simulink model "IEEE34_PQload"  (R2021b)
settings: Solver=ode4  StartTime=0.0  StopTime=5  FixedStep=50e-6  RelTol=1e-3
PreLoadFcn:
  | pGain = 0.05; % Gain of random perturbation (pu)
  | pGainAP = 0.01; % Gain of sinusoidal active power variation (pu)
  | pGainRP = 0.01; % Gain of sinusoidal reactive power variation (pu)
  | pFreqAP = 0.03; % Frequency of sinusoidal active power variation (Hz)
  | pFreqRP = 0.03; % Frequency of sinusoidal reactive power variation (Hz)
  | 
  | init_IEEE34nodetestfeeder;
InitFcn:
  | pGain = 0.05; % Gain of random perturbation (pu)
  | pGainAP = 0.01; % Gain of sinusoidal active power variation (pu)
  | pGainRP = 0.01; % Gain of sinusoidal reactive power variation (pu)
  | pFreqAP = 0.03; % Frequency of sinusoidal active power variation (Hz)
  | pFreqRP = 0.03; % Frequency of sinusoidal reactive power variation (Hz)
  | 
  | init_IEEE34nodetestfeeder;
values from neighbouring files (symbols this model uses):
  fNom = f    (= 60)    [init_IEEE34nodetestfeeder.m]
  loadcoeff = 1.0    (= 1)    [init_IEEE34nodetestfeeder.m]
  Pbase = 500e3    (= 500000)    [init_IEEE34nodetestfeeder.m]
  Ts = 50e-6    (= 5e-05)    [init_IEEE34nodetestfeeder.m]
  vNomMV = VsubL    (= 24900)    [init_IEEE34nodetestfeeder.m]
  VsubL = 24.9e3    (= 24900)    [init_IEEE34nodetestfeeder.m]
undefined symbols (not defined in the file or in its folder): find_system
libraries: spsSeriesRLCBranchLib x330, spsGroundLib x242, LoadLib x88, spsThreePhaseVIMeasurementLib x37, spsMutualInductanceLib x24, spsVoltageMeasurementLib x18, spsCurrentMeasurementLib x12, spsOnDelayLib x12, spsRMSLib x8, spsLinearTransformerLib x6, spsControlledCurrentSourceLib x6, spsControlledVoltageSourceLib x6
(part 6 of 8)

== system IEEE34_PQload/SM_IEEE34/Regulator 2 ==
  Mux : Mux  Inputs=3
  Single Phase SVR_A : Subsystem  LoadFcn=find_system(gcs,'FollowLinks', 'on', 'LookUnderMasks', 'all');  mask(Single-Phase OLTC){pNom=5e6/3, fNom=60, vNom=24.9e3/sqrt(3), ctRatio=100, ptRatio=120, DeltaU=0.00625, TapMinMax=[-16 16], InitialTap=-13, TapSelectionTime=0.2, RegulatorOn=off, Regulator=[124/120  2/120  0.2], Comp=[2.5 1.5]}
      mask prompts: pNom "Nominal Power (VA)"; fNom "Nominal Frequency (Hz)"; vNom "Nominal Voltage (Vrms)"; ctRatio "Primary CT Rating (A)"; ptRatio "PT Ratio"; DeltaU "Voltage Step Per Tap (pu)"; TapMinMax "Minimum and Maximum Tap Positions"; InitialTap "Initial Tap Position"; TapSelectionTime "Tap Selection Time (s)"; RegulatorOn "Voltage Regulator"; Regulator "Voltage Regulator [ Vref(pu) DeadBand(pu)  Delay(s)]"; Comp "Compensator Settings [R (V) X(V)]"
      mask help:
      | Models a single-phase On Load Tap Changer (OLTC). The single-phase primary of multi-tap winding is modeled with a Variable-Ratio Transformer block.
      |
      | The transformer voltage ratio U2/U1 (in pu) is given by:
      |                 U2/U1= 1/ (1+TapPosition*DeltaU)
      | Tap position 0 corresponds to nominal voltage ratio.
      |
      | When Voltage regulator is 'on',  voltage regulator asks for a tap change if:
      |                  abs(Vm-Vref)>DeadBand/2  during a time  t > Delay.
      |
      | where 'Vm' is voltage measured at regulating point and Vref is reference voltage.
      | With line drop compensation, Vm=Vsec-Isec(R+jX)
      mask init:
      | RegulatorVref=Regulator(1);
      | RegulatorDeadBand=Regulator(2);
      | RegulatorDelay=Regulator(3);
      | Rc=Comp(1);
      | Xc=Comp(2);
      mask TypeOptions RegulatorOn: off | on
      mask Callback RegulatorOn:
      | tempMaskVis=get_param(gcb,'MaskVisibilities');
      | if strcmp(get_param(gcb,'RegulatorOn'),'on')
      | 	tempMaskVis{11}='on';
      | 	set_param(gcb,'MaskVisibilities',tempMaskVis);
      | else
      | 	tempMaskVis{11}='off';
      | 	set_param(gcb,'MaskVisibilities',tempMaskVis);
      | end
      | if strcmp(get_param(gcb,'RegulatorOn'),'on')
      | 	tempMaskVis{12}='on';
      | 	set_param(gcb,'MaskVisibilities',tempMaskVis);
      | else
      | 	tempMaskVis{12}='off';
      | 	set_param(gcb,'MaskVisibilities',tempMaskVis);
      | end
      mask DialogControl Container8 Prompt: Setup
      mask DialogControl Container13 Prompt: Regulator Parameters
  Single Phase SVR_B : Subsystem  LoadFcn=find_system(gcs,'FollowLinks', 'on', 'LookUnderMasks', 'all');  mask(Single-Phase OLTC){pNom=5e6/3, fNom=60, vNom=24.9e3/sqrt(3), ctRatio=100, ptRatio=120, DeltaU=0.00625, TapMinMax=[-16 16], InitialTap=-11, TapSelectionTime=0.2, RegulatorOn=off, Regulator=[124/120  2/120  0.2], Comp=[2.5 1.5]}
      mask prompts: pNom "Nominal Power (VA)"; fNom "Nominal Frequency (Hz)"; vNom "Nominal Voltage (Vrms)"; ctRatio "Primary CT Rating (A)"; ptRatio "PT Ratio"; DeltaU "Voltage Step Per Tap (pu)"; TapMinMax "Minimum and Maximum Tap Positions"; InitialTap "Initial Tap Position"; TapSelectionTime "Tap Selection Time (s)"; RegulatorOn "Voltage Regulator"; Regulator "Voltage Regulator [ Vref(pu) DeadBand(pu)  Delay(s)]"; Comp "Compensator Settings [R (V) X(V)]"
      mask help:
      | Models a single-phase On Load Tap Changer (OLTC). The single-phase primary of multi-tap winding is modeled with a Variable-Ratio Transformer block.
      |
      | The transformer voltage ratio U2/U1 (in pu) is given by:
      |                 U2/U1= 1/ (1+TapPosition*DeltaU)
      | Tap position 0 corresponds to nominal voltage ratio.
      |
      | When Voltage regulator is 'on',  voltage regulator asks for a tap change if:
      |                  abs(Vm-Vref)>DeadBand/2  during a time  t > Delay.
      |
      | where 'Vm' is voltage measured at regulating point and Vref is reference voltage.
      | With line drop compensation, Vm=Vsec-Isec(R+jX)
      mask init:
      | RegulatorVref=Regulator(1);
      | RegulatorDeadBand=Regulator(2);
      | RegulatorDelay=Regulator(3);
      | Rc=Comp(1);
      | Xc=Comp(2);
      mask TypeOptions RegulatorOn: off | on
      mask Callback RegulatorOn:
      | tempMaskVis=get_param(gcb,'MaskVisibilities');
      | if strcmp(get_param(gcb,'RegulatorOn'),'on')
      | 	tempMaskVis{11}='on';
      | 	set_param(gcb,'MaskVisibilities',tempMaskVis);
      | else
      | 	tempMaskVis{11}='off';
      | 	set_param(gcb,'MaskVisibilities',tempMaskVis);
      | end
      | if strcmp(get_param(gcb,'RegulatorOn'),'on')
      | 	tempMaskVis{12}='on';
      | 	set_param(gcb,'MaskVisibilities',tempMaskVis);
      | else
      | 	tempMaskVis{12}='off';
      | 	set_param(gcb,'MaskVisibilities',tempMaskVis);
      | end
      mask DialogControl Container8 Prompt: Setup
      mask DialogControl Container13 Prompt: Regulator Parameters
  Single Phase SVR_C : Subsystem  LoadFcn=find_system(gcs,'FollowLinks', 'on', 'LookUnderMasks', 'all');  mask(Single-Phase OLTC){pNom=5e6/3, fNom=60, vNom=24.9e3/sqrt(3), ctRatio=100, ptRatio=120, DeltaU=0.00625, TapMinMax=[-16 16], InitialTap=-12, TapSelectionTime=0.2, RegulatorOn=off, Regulator=[124/120  2/120  0.2], Comp=[2.5 1.5]}
      mask prompts: pNom "Nominal Power (VA)"; fNom "Nominal Frequency (Hz)"; vNom "Nominal Voltage (Vrms)"; ctRatio "Primary CT Rating (A)"; ptRatio "PT Ratio"; DeltaU "Voltage Step Per Tap (pu)"; TapMinMax "Minimum and Maximum Tap Positions"; InitialTap "Initial Tap Position"; TapSelectionTime "Tap Selection Time (s)"; RegulatorOn "Voltage Regulator"; Regulator "Voltage Regulator [ Vref(pu) DeadBand(pu)  Delay(s)]"; Comp "Compensator Settings [R (V) X(V)]"
      mask help:
      | Models a single-phase On Load Tap Changer (OLTC). The single-phase primary of multi-tap winding is modeled with a Variable-Ratio Transformer block.
      |
      | The transformer voltage ratio U2/U1 (in pu) is given by:
      |                 U2/U1= 1/ (1+TapPosition*DeltaU)
      | Tap position 0 corresponds to nominal voltage ratio.
      |
      | When Voltage regulator is 'on',  voltage regulator asks for a tap change if:
      |                  abs(Vm-Vref)>DeadBand/2  during a time  t > Delay.
      |
      | where 'Vm' is voltage measured at regulating point and Vref is reference voltage.
      | With line drop compensation, Vm=Vsec-Isec(R+jX)
      mask init:
      | RegulatorVref=Regulator(1);
      | RegulatorDeadBand=Regulator(2);
      | RegulatorDelay=Regulator(3);
      | Rc=Comp(1);
      | Xc=Comp(2);
      mask TypeOptions RegulatorOn: off | on
      mask Callback RegulatorOn:
      | tempMaskVis=get_param(gcb,'MaskVisibilities');
      | if strcmp(get_param(gcb,'RegulatorOn'),'on')
      | 	tempMaskVis{11}='on';
      | 	set_param(gcb,'MaskVisibilities',tempMaskVis);
      | else
      | 	tempMaskVis{11}='off';
      | 	set_param(gcb,'MaskVisibilities',tempMaskVis);
      | end
      | if strcmp(get_param(gcb,'RegulatorOn'),'on')
      | 	tempMaskVis{12}='on';
      | 	set_param(gcb,'MaskVisibilities',tempMaskVis);
      | else
      | 	tempMaskVis{12}='off';
      | 	set_param(gcb,'MaskVisibilities',tempMaskVis);
      | end
      mask DialogControl Container8 Prompt: Setup
      mask DialogControl Container13 Prompt: Regulator Parameters
  A : PMIOPort  Side=Left
  a : PMIOPort  Port=2  Side=Right
  B : PMIOPort  Port=3  Side=Left
  b : PMIOPort  Port=4  Side=Right
  C : PMIOPort  Port=5  Side=Left
  c : PMIOPort  Port=6  Side=Right
  Tap : Outport
  wires:
  Single Phase SVR_A/1(Tap) -> Mux/1
  Single Phase SVR_B/1(Tap) -> Mux/2
  Single Phase SVR_C/1(Tap) -> Mux/3
  Mux/1 -> Tap/1
  connections:
  Single Phase SVR_A/RConn1 -- a/RConn1
  Single Phase SVR_A/LConn1 -- A/RConn1
  Single Phase SVR_B/LConn1 -- B/RConn1
  Single Phase SVR_B/RConn1 -- b/RConn1
  Single Phase SVR_C/LConn1 -- C/RConn1
  Single Phase SVR_C/RConn1 -- c/RConn1

== system IEEE34_PQload/SM_IEEE34/Spot 830 ==
  SinglePhase_PQLoadwithFeedback : LoadLib/SinglePhase_PQLoad  fnom=60  Vbase=VsubL  V0=1  S0=[10*1000*loadcoeff 5*1000*loadcoeff]/Pbase  PQext=off  Kpi=PI_values  BasePower=Pbase  n=[2 2]  T=[0 0 0 0]  Vmin=0.7  Freq_dep=on  FKpq=[0 0]  Ts=50e-6
  SinglePhase_PQLoadwithFeedback1 : LoadLib/SinglePhase_PQLoad  fnom=60  Vbase=VsubL  V0=1  S0=[10*1000*loadcoeff 5*1000*loadcoeff]/Pbase  PQext=off  Kpi=PI_values  BasePower=Pbase  n=[2 2]  T=[0 0 0 0]  Vmin=0.7  Freq_dep=on  FKpq=[0 0]  Ts=50e-6
  SinglePhase_PQLoadwithFeedback2 : LoadLib/SinglePhase_PQLoad  fnom=60  Vbase=VsubL  V0=1  S0=[25*1000*loadcoeff 10*1000*loadcoeff]/Pbase  PQext=off  Kpi=PI_values  BasePower=Pbase  n=[2 2]  T=[0 0 0 0]  Vmin=0.7  Freq_dep=on  FKpq=[0 0]  Ts=50e-6
  Terminator3 : Terminator
  Terminator4 : Terminator
  Terminator5 : Terminator
  A : PMIOPort  Side=Right
  B : PMIOPort  Port=2  Side=Right
  C : PMIOPort  Port=3  Side=Right
  wires:
  SinglePhase_PQLoadwithFeedback/1 -> Terminator3/1
  SinglePhase_PQLoadwithFeedback1/1 -> Terminator4/1
  SinglePhase_PQLoadwithFeedback2/1 -> Terminator5/1
  connections:
  SinglePhase_PQLoadwithFeedback/LConn1 -- SinglePhase_PQLoadwithFeedback2/LConn2 -- A/RConn1
  SinglePhase_PQLoadwithFeedback1/LConn1 -- SinglePhase_PQLoadwithFeedback/LConn2 -- B/RConn1
  SinglePhase_PQLoadwithFeedback2/LConn1 -- SinglePhase_PQLoadwithFeedback1/LConn2 -- C/RConn1

== system IEEE34_PQload/SM_IEEE34/Spot 840 ==
  Ground1 : spsGroundLib/Ground  LConnTagsString=a
  Ground2 : spsGroundLib/Ground  LConnTagsString=a
  Ground3 : spsGroundLib/Ground  LConnTagsString=a
  SinglePhase_PQLoadwithFeedback : LoadLib/SinglePhase_PQLoad  fnom=60  Vbase=VsubL/sqrt(3)  V0=1  S0=[9*1000*loadcoeff 7*1000*loadcoeff]/Pbase  PQext=off  Kpi=PI_values  BasePower=Pbase  n=[1 1]  T=[0 0 0 0]  Vmin=0.7  Freq_dep=on  FKpq=[0 0]  Ts=50e-6
  SinglePhase_PQLoadwithFeedback1 : LoadLib/SinglePhase_PQLoad  fnom=60  Vbase=VsubL/sqrt(3)  V0=1  S0=[9*1000*loadcoeff 7*1000*loadcoeff]/Pbase  PQext=off  Kpi=PI_values  BasePower=Pbase  n=[1 1]  T=[0 0 0 0]  Vmin=0.7  Freq_dep=on  FKpq=[0 0]  Ts=50e-6
  SinglePhase_PQLoadwithFeedback2 : LoadLib/SinglePhase_PQLoad  fnom=60  Vbase=VsubL/sqrt(3)  V0=1  S0=[9*1000*loadcoeff 7*1000*loadcoeff]/Pbase  PQext=off  Kpi=PI_values  BasePower=Pbase  n=[1 1]  T=[0 0 0 0]  Vmin=0.7  Freq_dep=on  FKpq=[0 0]  Ts=50e-6
  Terminator3 : Terminator
  Terminator4 : Terminator
  Terminator5 : Terminator
  A : PMIOPort  Side=Right
  B : PMIOPort  Port=2  Side=Right
  C : PMIOPort  Port=3  Side=Right
  wires:
  SinglePhase_PQLoadwithFeedback/1 -> Terminator3/1
  SinglePhase_PQLoadwithFeedback1/1 -> Terminator4/1
  SinglePhase_PQLoadwithFeedback2/1 -> Terminator5/1
  connections:
  SinglePhase_PQLoadwithFeedback/LConn2 -- Ground1/LConn1
  SinglePhase_PQLoadwithFeedback1/LConn2 -- Ground2/LConn1
  SinglePhase_PQLoadwithFeedback2/LConn2 -- Ground3/LConn1
  SinglePhase_PQLoadwithFeedback/LConn1 -- A/RConn1
  SinglePhase_PQLoadwithFeedback1/LConn1 -- B/RConn1
  SinglePhase_PQLoadwithFeedback2/LConn1 -- C/RConn1

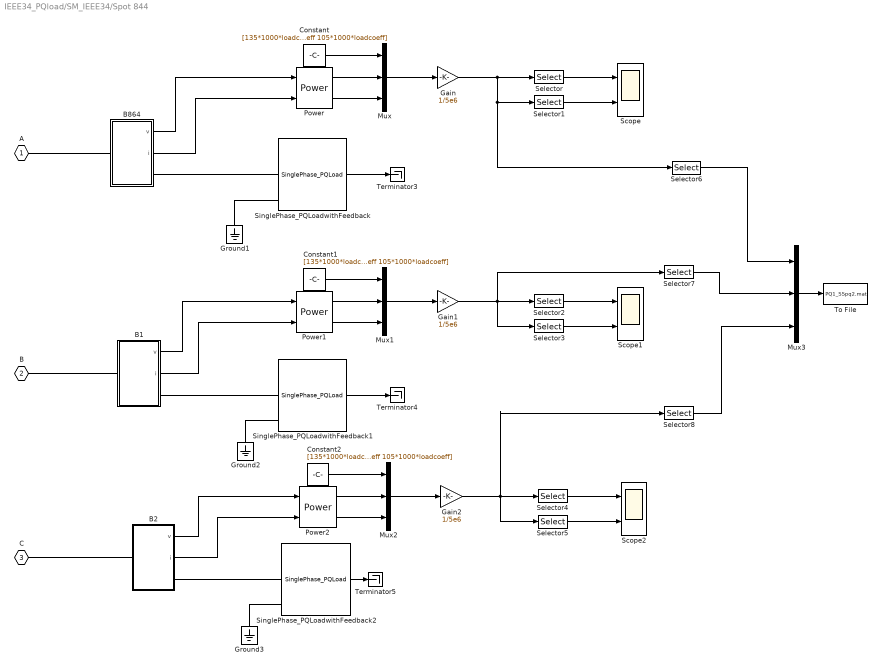
== system IEEE34_PQload/SM_IEEE34/Spot 844 ==
  B1 : Subsystem
  B2 : Subsystem
  B864 : Subsystem
  Constant : Constant  Value=[135*1000*loadcoeff 105*1000*loadcoeff]
  Constant1 : Constant  Value=[135*1000*loadcoeff 105*1000*loadcoeff]
  Constant2 : Constant  Value=[135*1000*loadcoeff 105*1000*loadcoeff]
  Gain : Gain  Gain=1/5e6
  Gain1 : Gain  Gain=1/5e6
  Gain2 : Gain  Gain=1/5e6
  Ground1 : spsGroundLib/Ground  LConnTagsString=a
  Ground2 : spsGroundLib/Ground  LConnTagsString=a
  Ground3 : spsGroundLib/Ground  LConnTagsString=a
  Mux{,1..3} (4 alike) : Mux  Inputs=3
  Power : spsPowerLib/Power  Freq=60  Vinit=[1, 0]  Iinit=[1, 0]  Ts=0
      settings: SourceProductBaseCode=PS
  Power1 : spsPowerLib/Power  Freq=60  Vinit=[1, 0]  Iinit=[1, 0]  Ts=0
      settings: SourceProductBaseCode=PS
  Power2 : spsPowerLib/Power  Freq=60  Vinit=[1, 0]  Iinit=[1, 0]  Ts=0
      settings: SourceProductBaseCode=PS
  Scope : Scope  NumInputPorts=2
  Scope1 : Scope  NumInputPorts=2
  Scope2 : Scope  NumInputPorts=2
  Selector : Selector  InputPortWidth=4  IndexOptions=Index vector (dialog)  Indices=[1 3]  OutputSizes=1
  Selector1 : Selector  InputPortWidth=4  IndexOptions=Index vector (dialog)  Indices=[2 4]  OutputSizes=1
  Selector2 : Selector  InputPortWidth=4  IndexOptions=Index vector (dialog)  Indices=[1 3]  OutputSizes=1
  Selector3 : Selector  InputPortWidth=4  IndexOptions=Index vector (dialog)  Indices=[2 4]  OutputSizes=1
  Selector4 : Selector  InputPortWidth=4  IndexOptions=Index vector (dialog)  Indices=[1 3]  OutputSizes=1
  Selector5 : Selector  InputPortWidth=4  IndexOptions=Index vector (dialog)  Indices=[2 4]  OutputSizes=1
  Selector6 : Selector  InputPortWidth=4  IndexOptions=Index vector (dialog)  Indices=[3 4]  OutputSizes=1
  Selector7 : Selector  InputPortWidth=4  IndexOptions=Index vector (dialog)  Indices=[3 4]  OutputSizes=1
  Selector8 : Selector  InputPortWidth=4  IndexOptions=Index vector (dialog)  Indices=[3 4]  OutputSizes=1
  SinglePhase_PQLoadwithFeedback : LoadLib/SinglePhase_PQLoad  fnom=60  Vbase=VsubL/sqrt(3)  V0=1  S0=[135*1000*loadcoeff 105*1000*loadcoeff]/Pbase  PQext=off  Kpi=PI_values  BasePower=Pbase  n=[2 2]  T=[0 0 0 0]  Vmin=0.7  Freq_dep=on  FKpq=[0 0]  Ts=50e-6
  SinglePhase_PQLoadwithFeedback1 : LoadLib/SinglePhase_PQLoad  fnom=60  Vbase=VsubL/sqrt(3)  V0=1  S0=[135*1000*loadcoeff 105*1000*loadcoeff]/Pbase  PQext=off  Kpi=PI_values  BasePower=Pbase  n=[2 2]  T=[0 0 0 0]  Vmin=0.7  Freq_dep=on  FKpq=[0 0]  Ts=50e-6
  SinglePhase_PQLoadwithFeedback2 : LoadLib/SinglePhase_PQLoad  fnom=60  Vbase=VsubL/sqrt(3)  V0=1  S0=[135*1000*loadcoeff 105*1000*loadcoeff]/Pbase  PQext=off  Kpi=PI_values  BasePower=Pbase  n=[2 2]  T=[0 0 0 0]  Vmin=0.7  Freq_dep=on  FKpq=[0 0]  Ts=50e-6
  Terminator3 : Terminator
  Terminator4 : Terminator
  Terminator5 : Terminator
  To File : ToFile  Filename=PQ1_SSpq2.mat  MatrixName=PQ1_SSpq2
  A : PMIOPort  Side=Right
  B : PMIOPort  Port=2  Side=Right
  C : PMIOPort  Port=3  Side=Right
  wires:
  SinglePhase_PQLoadwithFeedback/1 -> Terminator3/1
  SinglePhase_PQLoadwithFeedback1/1 -> Terminator4/1
  SinglePhase_PQLoadwithFeedback2/1 -> Terminator5/1
  Constant/1 -> Mux/1
  Selector1/1 -> Scope/2
  Power/1 -> Mux/2
  Gain/1 -> Selector6/1, Selector1/1, Selector/1
  Selector/1 -> Scope/1
  Power/2 -> Mux/3
  Mux/1 -> Gain/1
  B864/1(v) -> Power/1
  B864/2(i) -> Power/2
  Constant1/1 -> Mux1/1
  Selector3/1 -> Scope1/2
  Power1/1 -> Mux1/2
  Selector2/1 -> Scope1/1
  Power1/2 -> Mux1/3
  Mux1/1 -> Gain1/1
  B1/1(v) -> Power1/1
  B1/2(i) -> Power1/2
  Constant2/1 -> Mux2/1
  Selector5/1 -> Scope2/2
  Power2/1 -> Mux2/2
  Selector4/1 -> Scope2/1
  Power2/2 -> Mux2/3
  Mux2/1 -> Gain2/1
  B2/1(v) -> Power2/1
  B2/2(i) -> Power2/2
  Mux3/1 -> To File/1
  Gain1/1 -> Selector7/1, Selector3/1, Selector2/1
  Gain2/1 -> Selector5/1, Selector8/1, Selector4/1
  Selector6/1 -> Mux3/1
  Selector7/1 -> Mux3/2
  Selector8/1 -> Mux3/3
  connections:
  SinglePhase_PQLoadwithFeedback/LConn2 -- Ground1/LConn1
  SinglePhase_PQLoadwithFeedback1/LConn2 -- Ground2/LConn1
  SinglePhase_PQLoadwithFeedback2/LConn2 -- Ground3/LConn1
  B864/RConn1 -- SinglePhase_PQLoadwithFeedback/LConn1
  A/RConn1 -- B864/LConn1
  B1/RConn1 -- SinglePhase_PQLoadwithFeedback1/LConn1
  B/RConn1 -- B1/LConn1
  B2/RConn1 -- SinglePhase_PQLoadwithFeedback2/LConn1
  C/RConn1 -- B2/LConn1

== system IEEE34_PQload/SM_IEEE34/Spot 848 ==
  SinglePhase_PQLoadwithFeedback : LoadLib/SinglePhase_PQLoad  fnom=60  Vbase=VsubL/sqrt(3)  V0=1  S0=[20*1000*loadcoeff 16*1000*loadcoeff]/Pbase  PQext=off  Kpi=PI_values  BasePower=Pbase  n=[0 0]  T=[0 0 0 0]  Vmin=0.7  Freq_dep=on  FKpq=[0 0]  Ts=50e-6
  SinglePhase_PQLoadwithFeedback1 : LoadLib/SinglePhase_PQLoad  fnom=60  Vbase=VsubL/sqrt(3)  V0=1  S0=[20*1000*loadcoeff 16*1000*loadcoeff]/Pbase  PQext=off  Kpi=PI_values  BasePower=Pbase  n=[0 0]  T=[0 0 0 0]  Vmin=0.7  Freq_dep=on  FKpq=[0 0]  Ts=50e-6
  SinglePhase_PQLoadwithFeedback2 : LoadLib/SinglePhase_PQLoad  fnom=60  Vbase=VsubL/sqrt(3)  V0=1  S0=[20*1000*loadcoeff 16*1000*loadcoeff]/Pbase  PQext=off  Kpi=PI_values  BasePower=Pbase  n=[0 0]  T=[0 0 0 0]  Vmin=0.7  Freq_dep=on  FKpq=[0 0]  Ts=50e-6
  Terminator1 : Terminator
  Terminator4 : Terminator
  Terminator5 : Terminator
  A : PMIOPort  Side=Right
  B : PMIOPort  Port=2  Side=Right
  C : PMIOPort  Port=3  Side=Right
  wires:
  SinglePhase_PQLoadwithFeedback/1 -> Terminator1/1
  SinglePhase_PQLoadwithFeedback1/1 -> Terminator4/1
  SinglePhase_PQLoadwithFeedback2/1 -> Terminator5/1
  connections:
  SinglePhase_PQLoadwithFeedback1/LConn1 -- SinglePhase_PQLoadwithFeedback/LConn2 -- B/RConn1
  SinglePhase_PQLoadwithFeedback/LConn1 -- SinglePhase_PQLoadwithFeedback2/LConn2 -- A/RConn1
  SinglePhase_PQLoadwithFeedback2/LConn1 -- SinglePhase_PQLoadwithFeedback1/LConn2 -- C/RConn1

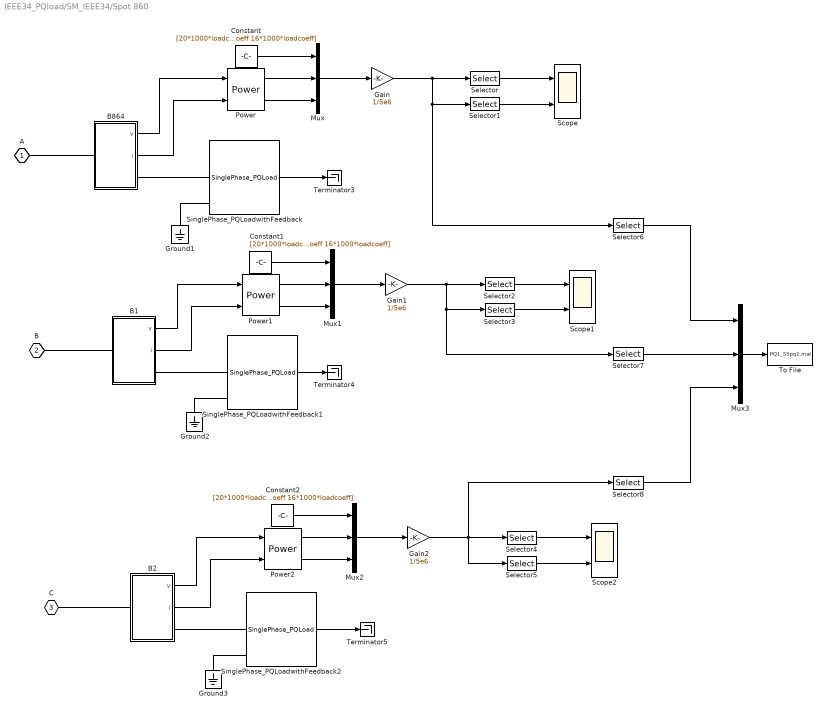
== system IEEE34_PQload/SM_IEEE34/Spot 860 ==
  B1 : Subsystem
  B2 : Subsystem
  B864 : Subsystem
  Constant : Constant  Value=[20*1000*loadcoeff 16*1000*loadcoeff]
  Constant1 : Constant  Value=[20*1000*loadcoeff 16*1000*loadcoeff]
  Constant2 : Constant  Value=[20*1000*loadcoeff 16*1000*loadcoeff]
  Gain : Gain  Gain=1/5e6
  Gain1 : Gain  Gain=1/5e6
  Gain2 : Gain  Gain=1/5e6
  Ground1 : spsGroundLib/Ground  LConnTagsString=a
  Ground2 : spsGroundLib/Ground  LConnTagsString=a
  Ground3 : spsGroundLib/Ground  LConnTagsString=a
  Mux{,1..3} (4 alike) : Mux  Inputs=3
  Power : spsPowerLib/Power  Freq=60  Vinit=[1, 0]  Iinit=[1, 0]  Ts=0
      settings: SourceProductBaseCode=PS
  Power1 : spsPowerLib/Power  Freq=60  Vinit=[1, 0]  Iinit=[1, 0]  Ts=0
      settings: SourceProductBaseCode=PS
  Power2 : spsPowerLib/Power  Freq=60  Vinit=[1, 0]  Iinit=[1, 0]  Ts=0
      settings: SourceProductBaseCode=PS
  Scope : Scope  NumInputPorts=2
  Scope1 : Scope  NumInputPorts=2
  Scope2 : Scope  NumInputPorts=2
  Selector : Selector  InputPortWidth=4  IndexOptions=Index vector (dialog)  Indices=[1 3]  OutputSizes=1
  Selector1 : Selector  InputPortWidth=4  IndexOptions=Index vector (dialog)  Indices=[2 4]  OutputSizes=1
  Selector2 : Selector  InputPortWidth=4  IndexOptions=Index vector (dialog)  Indices=[1 3]  OutputSizes=1
  Selector3 : Selector  InputPortWidth=4  IndexOptions=Index vector (dialog)  Indices=[2 4]  OutputSizes=1
  Selector4 : Selector  InputPortWidth=4  IndexOptions=Index vector (dialog)  Indices=[1 3]  OutputSizes=1
  Selector5 : Selector  InputPortWidth=4  IndexOptions=Index vector (dialog)  Indices=[2 4]  OutputSizes=1
  Selector6 : Selector  InputPortWidth=4  IndexOptions=Index vector (dialog)  Indices=[3 4]  OutputSizes=1
  Selector7 : Selector  InputPortWidth=4  IndexOptions=Index vector (dialog)  Indices=[3 4]  OutputSizes=1
  Selector8 : Selector  InputPortWidth=4  IndexOptions=Index vector (dialog)  Indices=[3 4]  OutputSizes=1
  SinglePhase_PQLoadwithFeedback : LoadLib/SinglePhase_PQLoad  fnom=60  Vbase=VsubL/sqrt(3)  V0=1  S0=[20*1000*loadcoeff 16*1000*loadcoeff]/Pbase  PQext=off  Kpi=PI_values  BasePower=Pbase  n=[0 0]  T=[0 0 0 0]  Vmin=0.7  Freq_dep=on  FKpq=[0 0]  Ts=50e-6
  SinglePhase_PQLoadwithFeedback1 : LoadLib/SinglePhase_PQLoad  fnom=60  Vbase=VsubL/sqrt(3)  V0=1  S0=[20*1000*loadcoeff 16*1000*loadcoeff]/Pbase  PQext=off  Kpi=PI_values  BasePower=Pbase  n=[0 0]  T=[0 0 0 0]  Vmin=0.7  Freq_dep=on  FKpq=[0 0]  Ts=50e-6
  SinglePhase_PQLoadwithFeedback2 : LoadLib/SinglePhase_PQLoad  fnom=60  Vbase=VsubL/sqrt(3)  V0=1  S0=[20*1000*loadcoeff 16*1000*loadcoeff]/Pbase  PQext=off  Kpi=PI_values  BasePower=Pbase  n=[0 0]  T=[0 0 0 0]  Vmin=0.7  Freq_dep=on  FKpq=[0 0]  Ts=50e-6
  Terminator3 : Terminator
  Terminator4 : Terminator
  Terminator5 : Terminator
  To File : ToFile  Filename=PQ1_SSpq1.mat  MatrixName=PQ1_SSpq1
  A : PMIOPort  Side=Right
  B : PMIOPort  Port=2  Side=Right
  C : PMIOPort  Port=3  Side=Right
  wires:
  SinglePhase_PQLoadwithFeedback/1 -> Terminator3/1
  SinglePhase_PQLoadwithFeedback1/1 -> Terminator4/1
  SinglePhase_PQLoadwithFeedback2/1 -> Terminator5/1
  Constant/1 -> Mux/1
  Selector1/1 -> Scope/2
  Power/1 -> Mux/2
  Gain/1 -> Selector6/1, Selector1/1, Selector/1
  Selector/1 -> Scope/1
  Power/2 -> Mux/3
  Mux/1 -> Gain/1
  B864/1(v) -> Power/1
  B864/2(i) -> Power/2
  Mux1/1 -> Gain1/1
  Power1/2 -> Mux1/3
  Selector2/1 -> Scope1/1
  Gain1/1 -> Selector2/1, Selector7/1, Selector3/1
  Power1/1 -> Mux1/2
  Selector3/1 -> Scope1/2
  Constant1/1 -> Mux1/1
  B1/1(v) -> Power1/1
  B1/2(i) -> Power1/2
  Constant2/1 -> Mux2/1
  Selector5/1 -> Scope2/2
  Power2/1 -> Mux2/2
  Gain2/1 -> Selector8/1, Selector5/1, Selector4/1
  Selector4/1 -> Scope2/1
  Power2/2 -> Mux2/3
  Mux2/1 -> Gain2/1
  B2/1(v) -> Power2/1
  B2/2(i) -> Power2/2
  Mux3/1 -> To File/1
  Selector7/1 -> Mux3/2
  Selector8/1 -> Mux3/3
  Selector6/1 -> Mux3/1
  connections:
  SinglePhase_PQLoadwithFeedback/LConn2 -- Ground1/LConn1
  SinglePhase_PQLoadwithFeedback1/LConn2 -- Ground2/LConn1
  SinglePhase_PQLoadwithFeedback2/LConn2 -- Ground3/LConn1
  B864/RConn1 -- SinglePhase_PQLoadwithFeedback/LConn1
  A/RConn1 -- B864/LConn1
  B1/RConn1 -- SinglePhase_PQLoadwithFeedback1/LConn1
  B/RConn1 -- B1/LConn1
  B2/RConn1 -- SinglePhase_PQLoadwithFeedback2/LConn1
  C/RConn1 -- B2/LConn1

== system IEEE34_PQload/SM_IEEE34/Spot 890 ==
  SinglePhase_PQLoadwithFeedback : LoadLib/SinglePhase_PQLoad  fnom=60  Vbase=VxfmL  V0=1  S0=[150*1000*loadcoeff 75*1000*loadcoeff]/Pbase  PQext=off  Kpi=PI_values  BasePower=Pbase  n=[1 1]  T=[0 0 0 0]  Vmin=0.7  Freq_dep=on  FKpq=[0 0]  Ts=50e-6
  SinglePhase_PQLoadwithFeedback1 : LoadLib/SinglePhase_PQLoad  fnom=60  Vbase=VxfmL  V0=1  S0=[150*1000*loadcoeff 75*1000*loadcoeff]/Pbase  PQext=off  Kpi=PI_values  BasePower=Pbase  n=[1 1]  T=[0 0 0 0]  Vmin=0.7  Freq_dep=on  FKpq=[0 0]  Ts=50e-6
  SinglePhase_PQLoadwithFeedback2 : LoadLib/SinglePhase_PQLoad  fnom=60  Vbase=VxfmL  V0=1  S0=[150*1000*loadcoeff 75*1000*loadcoeff]/Pbase  PQext=off  Kpi=PI_values  BasePower=Pbase  n=[1 1]  T=[0 0 0 0]  Vmin=0.7  Freq_dep=on  FKpq=[0 0]  Ts=50e-6
  Terminator3 : Terminator
  Terminator4 : Terminator
  Terminator5 : Terminator
  A : PMIOPort  Side=Right
  B : PMIOPort  Port=2  Side=Right
  C : PMIOPort  Port=3  Side=Right
  wires:
  SinglePhase_PQLoadwithFeedback/1 -> Terminator3/1
  SinglePhase_PQLoadwithFeedback1/1 -> Terminator4/1
  SinglePhase_PQLoadwithFeedback2/1 -> Terminator5/1
  connections:
  SinglePhase_PQLoadwithFeedback/LConn1 -- SinglePhase_PQLoadwithFeedback2/LConn2 -- A/RConn1
  SinglePhase_PQLoadwithFeedback1/LConn1 -- SinglePhase_PQLoadwithFeedback/LConn2 -- B/RConn1
  SinglePhase_PQLoadwithFeedback2/LConn1 -- SinglePhase_PQLoadwithFeedback1/LConn2 -- C/RConn1

== system IEEE34_PQload/SM_IEEE34/Regulator 1/Single Phase SVR_A ==
  Line Drop Compensator : Subsystem
  Transformer with Taps : Subsystem
  Voltage Regulator Control : Subsystem
  S : PMIOPort  Tag=PMCPort  Side=Left
  L : PMIOPort  Tag=PMCPort  Port=2  Side=Right
  Tap : Outport  VectorParamsAs1DForOutWhenUnconnected=off
  tag scope: Vr1a=global
  wires:
  Transformer with Taps/2(Vsec) -> Line Drop Compensator/2(Vsec)
  Transformer with Taps/1(Isec) -> Line Drop Compensator/1(Isec)
  Voltage Regulator Control/1(N) -> Transformer with Taps/1(N)
  Voltage Regulator Control/2(Tap) -> Tap/1
  Line Drop Compensator/1(Vm) -> [Vr1a], Voltage Regulator Control/1(Vm)
  connections:
  S/RConn1 -- Transformer with Taps/LConn1
  Transformer with Taps/RConn1 -- L/RConn1

== system IEEE34_PQload/SM_IEEE34/Regulator 1/Single Phase SVR_B ==
  Line Drop Compensator : Subsystem
  Transformer with Taps : Subsystem
  Voltage Regulator Control : Subsystem
  S : PMIOPort  Tag=PMCPort  Side=Left
  L : PMIOPort  Tag=PMCPort  Port=2  Side=Right
  Tap : Outport  VectorParamsAs1DForOutWhenUnconnected=off
  tag scope: Vr1b=global
  wires:
  Line Drop Compensator/1(Vm) -> Voltage Regulator Control/1(Vm), [Vr1b]
  Voltage Regulator Control/2(Tap) -> Tap/1
  Voltage Regulator Control/1(N) -> Transformer with Taps/1(N)
  Transformer with Taps/1(Isec) -> Line Drop Compensator/1(Isec)
  Transformer with Taps/2(Vsec) -> Line Drop Compensator/2(Vsec)
  connections:
  Transformer with Taps/RConn1 -- L/RConn1
  S/RConn1 -- Transformer with Taps/LConn1

== system IEEE34_PQload/SM_IEEE34/Regulator 1/Single Phase SVR_C ==
  Line Drop Compensator : Subsystem
  Transformer with Taps : Subsystem
  Voltage Regulator Control : Subsystem
  S : PMIOPort  Tag=PMCPort  Side=Left
  L : PMIOPort  Tag=PMCPort  Port=2  Side=Right
  Tap : Outport  VectorParamsAs1DForOutWhenUnconnected=off
  tag scope: Vr1c=global
  wires:
  Transformer with Taps/2(Vsec) -> Line Drop Compensator/2(Vsec)
  Transformer with Taps/1(Isec) -> Line Drop Compensator/1(Isec)
  Voltage Regulator Control/1(N) -> Transformer with Taps/1(N)
  Voltage Regulator Control/2(Tap) -> Tap/1
  Line Drop Compensator/1(Vm) -> [Vr1c], Voltage Regulator Control/1(Vm)
  connections:
  S/RConn1 -- Transformer with Taps/LConn1
  Transformer with Taps/RConn1 -- L/RConn1

== system IEEE34_PQload/SM_IEEE34/Regulator 2/Single Phase SVR_A ==
  Line Drop Compensator : Subsystem
  Transformer with Taps : Subsystem
  Voltage Regulator Control : Subsystem
  S : PMIOPort  Tag=PMCPort  Side=Left
  L : PMIOPort  Tag=PMCPort  Port=2  Side=Right
  Tap : Outport  VectorParamsAs1DForOutWhenUnconnected=off
  tag scope: Vr2a=global
  wires:
  Transformer with Taps/2(Vsec) -> Line Drop Compensator/2(Vsec)
  Transformer with Taps/1(Isec) -> Line Drop Compensator/1(Isec)
  Voltage Regulator Control/1(N) -> Transformer with Taps/1(N)
  Voltage Regulator Control/2(Tap) -> Tap/1
  Line Drop Compensator/1(Vm) -> Voltage Regulator Control/1(Vm), [Vr2a]
  connections:
  S/RConn1 -- Transformer with Taps/LConn1
  Transformer with Taps/RConn1 -- L/RConn1

== system IEEE34_PQload/SM_IEEE34/Regulator 2/Single Phase SVR_B ==
  Line Drop Compensator : Subsystem
  Transformer with Taps : Subsystem
  Voltage Regulator Control : Subsystem
  S : PMIOPort  Tag=PMCPort  Side=Left
  L : PMIOPort  Tag=PMCPort  Port=2  Side=Right
  Tap : Outport  VectorParamsAs1DForOutWhenUnconnected=off
  tag scope: Vr2b=global
  wires:
  Line Drop Compensator/1(Vm) -> [Vr2b], Voltage Regulator Control/1(Vm)
  Voltage Regulator Control/2(Tap) -> Tap/1
  Voltage Regulator Control/1(N) -> Transformer with Taps/1(N)
  Transformer with Taps/1(Isec) -> Line Drop Compensator/1(Isec)
  Transformer with Taps/2(Vsec) -> Line Drop Compensator/2(Vsec)
  connections:
  Transformer with Taps/RConn1 -- L/RConn1
  S/RConn1 -- Transformer with Taps/LConn1

== system IEEE34_PQload/SM_IEEE34/Regulator 2/Single Phase SVR_C ==
  Line Drop Compensator : Subsystem
  Transformer with Taps : Subsystem
  Voltage Regulator Control : Subsystem
  S : PMIOPort  Tag=PMCPort  Side=Left
  L : PMIOPort  Tag=PMCPort  Port=2  Side=Right
  Tap : Outport  VectorParamsAs1DForOutWhenUnconnected=off
  tag scope: Vr2c=global
  wires:
  Transformer with Taps/2(Vsec) -> Line Drop Compensator/2(Vsec)
  Transformer with Taps/1(Isec) -> Line Drop Compensator/1(Isec)
  Voltage Regulator Control/1(N) -> Transformer with Taps/1(N)
  Voltage Regulator Control/2(Tap) -> Tap/1
  Line Drop Compensator/1(Vm) -> Voltage Regulator Control/1(Vm), [Vr2c]
  connections:
  S/RConn1 -- Transformer with Taps/LConn1
  Transformer with Taps/RConn1 -- L/RConn1

== system IEEE34_PQload/SM_IEEE34/Spot 844/B1 ==
  Ground : spsGroundLib/Ground  LConnTagsString=a
  I : spsCurrentMeasurementLib/Current Measurement  PhasorSimulation=off  OutputType=Complex  PSBequivalent=0
  V : spsVoltageMeasurementLib/Voltage Measurement  PhasorSimulation=off  OutputType=Complex  PSBequivalent=0
  A : PMIOPort  Side=Left
  B : PMIOPort  Port=2  Side=Right
  v : Outport
  i : Outport  Port=2
  wires:
  I/1 -> i/1
  V/1 -> v/1
  connections:
  B/RConn1 -- I/RConn1
  Ground/LConn1 -- V/LConn2
  A/RConn1 -- I/LConn1 -- V/LConn1

== system IEEE34_PQload/SM_IEEE34/Spot 844/B2 ==
  Ground : spsGroundLib/Ground  LConnTagsString=a
  I : spsCurrentMeasurementLib/Current Measurement  PhasorSimulation=off  OutputType=Complex  PSBequivalent=0
  V : spsVoltageMeasurementLib/Voltage Measurement  PhasorSimulation=off  OutputType=Complex  PSBequivalent=0
  A : PMIOPort  Side=Left
  B : PMIOPort  Port=2  Side=Right
  v : Outport
  i : Outport  Port=2
  wires:
  V/1 -> v/1
  I/1 -> i/1
  connections:
  V/LConn1 -- I/LConn1 -- A/RConn1
  Ground/LConn1 -- V/LConn2
  B/RConn1 -- I/RConn1

== system IEEE34_PQload/SM_IEEE34/Spot 844/B864 ==
  Ground : spsGroundLib/Ground  LConnTagsString=a
  I : spsCurrentMeasurementLib/Current Measurement  PhasorSimulation=off  OutputType=Complex  PSBequivalent=0
  V : spsVoltageMeasurementLib/Voltage Measurement  PhasorSimulation=off  OutputType=Complex  PSBequivalent=0
  A : PMIOPort  Side=Left
  B : PMIOPort  Port=2  Side=Right
  v : Outport
  i : Outport  Port=2
  wires:
  V/1 -> v/1
  I/1 -> i/1
  connections:
  V/LConn1 -- I/LConn1 -- A/RConn1
  Ground/LConn1 -- V/LConn2
  B/RConn1 -- I/RConn1

== system IEEE34_PQload/SM_IEEE34/Spot 860/B1 ==
  Ground : spsGroundLib/Ground  LConnTagsString=a
  I : spsCurrentMeasurementLib/Current Measurement  PhasorSimulation=off  OutputType=Complex  PSBequivalent=0
  V : spsVoltageMeasurementLib/Voltage Measurement  PhasorSimulation=off  OutputType=Complex  PSBequivalent=0
  A : PMIOPort  Side=Left
  B : PMIOPort  Port=2  Side=Right
  v : Outport
  i : Outport  Port=2
  wires:
  I/1 -> i/1
  V/1 -> v/1
  connections:
  B/RConn1 -- I/RConn1
  Ground/LConn1 -- V/LConn2
  A/RConn1 -- I/LConn1 -- V/LConn1

== system IEEE34_PQload/SM_IEEE34/Spot 860/B2 ==
  Ground : spsGroundLib/Ground  LConnTagsString=a
  I : spsCurrentMeasurementLib/Current Measurement  PhasorSimulation=off  OutputType=Complex  PSBequivalent=0
  V : spsVoltageMeasurementLib/Voltage Measurement  PhasorSimulation=off  OutputType=Complex  PSBequivalent=0
  A : PMIOPort  Side=Left
  B : PMIOPort  Port=2  Side=Right
  v : Outport
  i : Outport  Port=2
  wires:
  V/1 -> v/1
  I/1 -> i/1
  connections:
  V/LConn1 -- I/LConn1 -- A/RConn1
  Ground/LConn1 -- V/LConn2
  B/RConn1 -- I/RConn1

== system IEEE34_PQload/SM_IEEE34/Spot 860/B864 ==
  Ground : spsGroundLib/Ground  LConnTagsString=a
  I : spsCurrentMeasurementLib/Current Measurement  PhasorSimulation=off  OutputType=Complex  PSBequivalent=0
  V : spsVoltageMeasurementLib/Voltage Measurement  PhasorSimulation=off  OutputType=Complex  PSBequivalent=0
  A : PMIOPort  Side=Left
  B : PMIOPort  Port=2  Side=Right
  v : Outport
  i : Outport  Port=2
  wires:
  V/1 -> v/1
  I/1 -> i/1
  connections:
  V/LConn1 -- I/LConn1 -- A/RConn1
  Ground/LConn1 -- V/LConn2
  B/RConn1 -- I/RConn1

== system IEEE34_PQload/SM_IEEE34/Regulator 1/Single Phase SVR_A/Line Drop Compensator ==
  note: Vm=Vsec-Isec(Rc+jXc)
  Isec : Inport
  Vsec : Inport  Port=2
  "        " : spsLinearTransformerLib/Linear Transformer  UNITS=SI  NominalPower=[pNom fNom]  winding1=[vNom/ptRatio 1e-7 1e-8]  winding2=[vNom/ptRatio 1e-7 1e-8]  ThreeWindings=off  winding3=[3.15e+005 0.7938 0.084225]  RmLm=[1e5 1e5]  Measurements=None  DataType=on
  "CTS  " : spsControlledCurrentSourceLib/Controlled Current Source  Initialize=on  Source_Type=AC  Amplitude=0  Phase=0  Frequency=0  Measurements=None
  "PTS  " : spsControlledVoltageSourceLib/Controlled Voltage Source  Initialize=on  Source_Type=AC  Amplitude=0  Phase=0  Frequency=0  Measurements=None
  RMS : spsRMSLib/RMS  TrueRMS=on  Freq=60  RMSInit=120  Ts=0
  Raux : spsSeriesRLCBranchLib/Series RLC Branch  LConnTagsString=__new0  RConnTagsString=__new0  BranchType=R  Resistance=1e2  Inductance=1.6 / (120*pi)  SetiL0=off  InitialCurrent=0  Capacitance=1e-6  Setx0=off  InitialVoltage=0  Measurements=None
  Rc+jXc : spsSeriesRLCBranchLib/Series RLC Branch  LConnTagsString=__new0  RConnTagsString=__new0  BranchType=RL  Resistance=Rc  Inductance=Xc / (2*pi*fNom)  SetiL0=off  InitialCurrent=0  Capacitance=1e-6  Setx0=off  InitialVoltage=0  Measurements=None
  VRelay : spsVoltageMeasurementLib/Voltage Measurement  PhasorSimulation=off  OutputType=Complex  PSBequivalent=0
  Vm : Outport
  wires:
  Vsec/1 -> "PTS  "/1
  Isec/1 -> "CTS  "/1
  VRelay/1 -> RMS/1
  RMS/1 -> Vm/1
  connections:
  VRelay/LConn2 -- "PTS  "/LConn1
  "        "/LConn2 -- "CTS  "/LConn1 -- Raux/RConn1 -- Rc+jXc/RConn1
  "CTS  "/RConn1 -- "        "/LConn1 -- Rc+jXc/LConn1 -- Raux/LConn1
  "        "/RConn2 -- VRelay/LConn1
  "PTS  "/RConn1 -- "        "/RConn1

== system IEEE34_PQload/SM_IEEE34/Regulator 1/Single Phase SVR_A/Transformer with Taps ==
  note: Isec on CT Ratio base
  note: Vsec on Pt Ratio base
  N : Inport
  "    " : Gain  Gain=1/ptRatio
  " 1" : Gain  Gain=1/ctRatio
  CT : spsCurrentMeasurementLib/Current Measurement  PhasorSimulation=off  OutputType=Complex  PSBequivalent=0
  Display : Display
  Display1 : Display
  Ground1 : spsGroundLib/Ground  LConnTagsString=a
  Ground2 : spsGroundLib/Ground  LConnTagsString=a
  Ground3 : spsGroundLib/Ground  LConnTagsString=a
  Memory : Memory
  Memory1 : Memory
  PT : spsVoltageMeasurementLib/Voltage Measurement  PhasorSimulation=off  OutputType=Complex  PSBequivalent=0
  "Variable-Ratio Transformer " : spsVariableRatioTransformerLib/Variable-Ratio Transformer
      settings: SourceProductBaseCode=PS
  rs : spsSeriesRLCBranchLib/Series RLC Branch  LConnTagsString=__new0  RConnTagsString=__new0  BranchType=R  Resistance=1e-6  Inductance=1e-3  SetiL0=off  InitialCurrent=0  Capacitance=1e-6  Setx0=off  InitialVoltage=0  Measurements=None
  L : PMIOPort  Tag=PMCPort  Side=Right
  S : PMIOPort  Port=2  Side=Left
  Isec : Outport
  Vsec : Outport  Port=2
  wires:
  Memory/1 -> Isec/1
  Memory1/1 -> Vsec/1
  N/1 -> "Variable-Ratio Transformer "/1
  " 1"/1 -> Memory/1
  CT/1 -> Display/1, " 1"/1
  PT/1 -> Display1/1, "    "/1
  "    "/1 -> Memory1/1
  connections:
  S/RConn1 -- "Variable-Ratio Transformer "/LConn1
  Ground2/LConn1 -- "Variable-Ratio Transformer "/RConn2
  Ground3/LConn1 -- "Variable-Ratio Transformer "/LConn2
  "Variable-Ratio Transformer "/RConn1 -- rs/LConn1
  CT/RConn1 -- L/RConn1
  PT/LConn1 -- rs/RConn1 -- CT/LConn1
  PT/LConn2 -- Ground1/LConn1

== system IEEE34_PQload/SM_IEEE34/Regulator 1/Single Phase SVR_A/Voltage Regulator Control ==
  note: N= 1/ (1+TapPosition*DeltaU)
  Vm : Inport
  1 : Constant
  Constant : Constant  Value=RegulatorOn
  Constant5 : Constant
  Product : Product  Inputs=/*
  Sum : Sum
  Tap Changer Control : Subsystem  mask(Tap Changer Control){MinMaxTap=TapMinMax, InitialPosition=InitialTap, MecDelay=TapSelectionTime}
      mask prompts: MinMaxTap "Minimum and maximum tap number [ Min  Max ] :"; InitialPosition "Initial tap position"; MecDelay "Mechanical delay time"
      mask init:
      | if MecDelay<=0,
      | 	MecDelay=1/60;
      | end
  Voltage change per tap : Gain  Gain=DeltaU
  Voltage regulator : Subsystem  mask{Vref=RegulatorVref*120, DeadBand=RegulatorDeadBand*120, TimeDelay=RegulatorDelay}
      mask prompts: Vref "Vref (on 120v base)"; DeadBand "Deadband (on 120v base)"; TimeDelay "Time delay (s)"
  N : Outport
  Tap : Outport  Port=2
  wires:
  Vm/1 -> Voltage regulator/1(Vmes (pu))
  Product/1 -> N/1
  Constant/1 -> Voltage regulator/3(RegOn)
  Tap Changer Control/2(Ready) -> Voltage regulator/2(Ready)
  Voltage change per tap/1 -> Sum/2
  Constant5/1 -> Sum/1
  Voltage regulator/1(Up) -> Tap Changer Control/1("Up ")
  Tap Changer Control/1(TapNo) -> Voltage change per tap/1, Tap/1  "Tap"
  1/1 -> Product/2
  Sum/1 -> Product/1
  Voltage regulator/2(Down) -> Tap Changer Control/2("Down ")

== system IEEE34_PQload/SM_IEEE34/Regulator 1/Single Phase SVR_B/Line Drop Compensator ==
  note: Vm=Vsec-Isec(Rc+jXc)
  Isec : Inport
  Vsec : Inport  Port=2
  "        " : spsLinearTransformerLib/Linear Transformer  UNITS=SI  NominalPower=[pNom fNom]  winding1=[vNom/ptRatio 1e-7 1e-8]  winding2=[vNom/ptRatio 1e-7 1e-8]  ThreeWindings=off  winding3=[3.15e+005 0.7938 0.084225]  RmLm=[1e5 1e5]  Measurements=None  DataType=on
  "CTS  " : spsControlledCurrentSourceLib/Controlled Current Source  Initialize=on  Source_Type=AC  Amplitude=0  Phase=0  Frequency=0  Measurements=None
  "PTS  " : spsControlledVoltageSourceLib/Controlled Voltage Source  Initialize=on  Source_Type=AC  Amplitude=0  Phase=0  Frequency=0  Measurements=None
  RMS : spsRMSLib/RMS  TrueRMS=on  Freq=60  RMSInit=120  Ts=0
  Raux : spsSeriesRLCBranchLib/Series RLC Branch  LConnTagsString=__new0  RConnTagsString=__new0  BranchType=R  Resistance=1e2  Inductance=1.6 / (120*pi)  SetiL0=off  InitialCurrent=0  Capacitance=1e-6  Setx0=off  InitialVoltage=0  Measurements=None
  Rc+jXc : spsSeriesRLCBranchLib/Series RLC Branch  LConnTagsString=__new0  RConnTagsString=__new0  BranchType=RL  Resistance=Rc  Inductance=Xc / (2*pi*fNom)  SetiL0=off  InitialCurrent=0  Capacitance=1e-6  Setx0=off  InitialVoltage=0  Measurements=None
  VRelay : spsVoltageMeasurementLib/Voltage Measurement  PhasorSimulation=off  OutputType=Complex  PSBequivalent=0
  Vm : Outport
  wires:
  RMS/1 -> Vm/1
  VRelay/1 -> RMS/1
  Isec/1 -> "CTS  "/1
  Vsec/1 -> "PTS  "/1
  connections:
  "PTS  "/RConn1 -- "        "/RConn1
  "        "/RConn2 -- VRelay/LConn1
  Raux/LConn1 -- Rc+jXc/LConn1 -- "        "/LConn1 -- "CTS  "/RConn1
  Rc+jXc/RConn1 -- Raux/RConn1 -- "CTS  "/LConn1 -- "        "/LConn2
  VRelay/LConn2 -- "PTS  "/LConn1

== system IEEE34_PQload/SM_IEEE34/Regulator 1/Single Phase SVR_B/Transformer with Taps ==
  note: Vsec on Pt Ratio base
  note: Isec on CT Ratio base
  N : Inport
  "    " : Gain  Gain=1/ptRatio
  " 1" : Gain  Gain=1/ctRatio
  CT : spsCurrentMeasurementLib/Current Measurement  PhasorSimulation=off  OutputType=Complex  PSBequivalent=0
  Display : Display
  Display1 : Display
  Ground1 : spsGroundLib/Ground  LConnTagsString=a
  Ground2 : spsGroundLib/Ground  LConnTagsString=a
  Ground3 : spsGroundLib/Ground  LConnTagsString=a
  Memory : Memory
  Memory1 : Memory
  PT : spsVoltageMeasurementLib/Voltage Measurement  PhasorSimulation=off  OutputType=Complex  PSBequivalent=0
  "Variable-Ratio Transformer " : spsVariableRatioTransformerLib/Variable-Ratio Transformer
      settings: SourceProductBaseCode=PS
  rs : spsSeriesRLCBranchLib/Series RLC Branch  LConnTagsString=__new0  RConnTagsString=__new0  BranchType=R  Resistance=1e-6  Inductance=1e-3  SetiL0=off  InitialCurrent=0  Capacitance=1e-6  Setx0=off  InitialVoltage=0  Measurements=None
  L : PMIOPort  Tag=PMCPort  Side=Right
  S : PMIOPort  Port=2  Side=Left
  Isec : Outport
  Vsec : Outport  Port=2
  wires:
  "    "/1 -> Memory1/1
  PT/1 -> "    "/1, Display1/1
  CT/1 -> " 1"/1, Display/1
  " 1"/1 -> Memory/1
  N/1 -> "Variable-Ratio Transformer "/1
  Memory1/1 -> Vsec/1
  Memory/1 -> Isec/1
  connections:
  PT/LConn2 -- Ground1/LConn1
  CT/LConn1 -- rs/RConn1 -- PT/LConn1
  CT/RConn1 -- L/RConn1
  "Variable-Ratio Transformer "/RConn1 -- rs/LConn1
  Ground3/LConn1 -- "Variable-Ratio Transformer "/LConn2
  Ground2/LConn1 -- "Variable-Ratio Transformer "/RConn2
  S/RConn1 -- "Variable-Ratio Transformer "/LConn1

== system IEEE34_PQload/SM_IEEE34/Regulator 1/Single Phase SVR_B/Voltage Regulator Control ==
  note: N= 1/ (1+TapPosition*DeltaU)
  Vm : Inport
  1 : Constant
  Constant : Constant  Value=RegulatorOn
  Constant5 : Constant
  Product : Product  Inputs=/*
  Sum : Sum
  Tap Changer Control : Subsystem  mask(Tap Changer Control){MinMaxTap=TapMinMax, InitialPosition=InitialTap, MecDelay=TapSelectionTime}
      mask prompts: MinMaxTap "Minimum and maximum tap number [ Min  Max ] :"; InitialPosition "Initial tap position"; MecDelay "Mechanical delay time"
      mask init:
      | if MecDelay<=0,
      | 	MecDelay=1/60;
      | end
  Voltage change per tap : Gain  Gain=DeltaU
  Voltage regulator : Subsystem  mask{Vref=RegulatorVref*120, DeadBand=RegulatorDeadBand*120, TimeDelay=RegulatorDelay}
      mask prompts: Vref "Vref (on 120v base)"; DeadBand "Deadband (on 120v base)"; TimeDelay "Time delay (s)"
  N : Outport
  Tap : Outport  Port=2
  wires:
  Voltage regulator/2(Down) -> Tap Changer Control/2("Down ")
  Sum/1 -> Product/1
  1/1 -> Product/2
  Tap Changer Control/1(TapNo) -> Tap/1, Voltage change per tap/1  "Tap"
  Voltage regulator/1(Up) -> Tap Changer Control/1("Up ")
  Constant5/1 -> Sum/1
  Voltage change per tap/1 -> Sum/2
  Tap Changer Control/2(Ready) -> Voltage regulator/2(Ready)
  Constant/1 -> Voltage regulator/3(RegOn)
  Product/1 -> N/1
  Vm/1 -> Voltage regulator/1(Vmes (pu))

== system IEEE34_PQload/SM_IEEE34/Regulator 1/Single Phase SVR_C/Line Drop Compensator ==
  note: Vm=Vsec-Isec(Rc+jXc)
  Isec : Inport
  Vsec : Inport  Port=2
  "        " : spsLinearTransformerLib/Linear Transformer  UNITS=SI  NominalPower=[pNom fNom]  winding1=[vNom/ptRatio 1e-7 1e-8]  winding2=[vNom/ptRatio 1e-7 1e-8]  ThreeWindings=off  winding3=[3.15e+005 0.7938 0.084225]  RmLm=[1e5 1e5]  Measurements=None  DataType=on
  "CTS  " : spsControlledCurrentSourceLib/Controlled Current Source  Initialize=on  Source_Type=AC  Amplitude=0  Phase=0  Frequency=0  Measurements=None
  "PTS  " : spsControlledVoltageSourceLib/Controlled Voltage Source  Initialize=on  Source_Type=AC  Amplitude=0  Phase=0  Frequency=0  Measurements=None
  RMS : spsRMSLib/RMS  TrueRMS=on  Freq=60  RMSInit=120  Ts=0
  Raux : spsSeriesRLCBranchLib/Series RLC Branch  LConnTagsString=__new0  RConnTagsString=__new0  BranchType=R  Resistance=1e2  Inductance=1.6 / (120*pi)  SetiL0=off  InitialCurrent=0  Capacitance=1e-6  Setx0=off  InitialVoltage=0  Measurements=None
  Rc+jXc : spsSeriesRLCBranchLib/Series RLC Branch  LConnTagsString=__new0  RConnTagsString=__new0  BranchType=RL  Resistance=Rc  Inductance=Xc / (2*pi*fNom)  SetiL0=off  InitialCurrent=0  Capacitance=1e-6  Setx0=off  InitialVoltage=0  Measurements=None
  VRelay : spsVoltageMeasurementLib/Voltage Measurement  PhasorSimulation=off  OutputType=Complex  PSBequivalent=0
  Vm : Outport
  wires:
  Vsec/1 -> "PTS  "/1
  Isec/1 -> "CTS  "/1
  VRelay/1 -> RMS/1
  RMS/1 -> Vm/1
  connections:
  VRelay/LConn2 -- "PTS  "/LConn1
  "        "/LConn2 -- "CTS  "/LConn1 -- Raux/RConn1 -- Rc+jXc/RConn1
  "CTS  "/RConn1 -- "        "/LConn1 -- Rc+jXc/LConn1 -- Raux/LConn1
  "        "/RConn2 -- VRelay/LConn1
  "PTS  "/RConn1 -- "        "/RConn1

== system IEEE34_PQload/SM_IEEE34/Regulator 1/Single Phase SVR_C/Transformer with Taps ==
  note: Isec on CT Ratio base
  note: Vsec on Pt Ratio base
  N : Inport
  "    " : Gain  Gain=1/ptRatio
  " 1" : Gain  Gain=1/ctRatio
  CT : spsCurrentMeasurementLib/Current Measurement  PhasorSimulation=off  OutputType=Complex  PSBequivalent=0
  Display : Display
  Display1 : Display
  Ground1 : spsGroundLib/Ground  LConnTagsString=a
  Ground2 : spsGroundLib/Ground  LConnTagsString=a
  Ground3 : spsGroundLib/Ground  LConnTagsString=a
  Memory : Memory
  Memory1 : Memory
  PT : spsVoltageMeasurementLib/Voltage Measurement  PhasorSimulation=off  OutputType=Complex  PSBequivalent=0
  "Variable-Ratio Transformer " : spsVariableRatioTransformerLib/Variable-Ratio Transformer
      settings: SourceProductBaseCode=PS
  rs : spsSeriesRLCBranchLib/Series RLC Branch  LConnTagsString=__new0  RConnTagsString=__new0  BranchType=R  Resistance=1e-6  Inductance=1e-3  SetiL0=off  InitialCurrent=0  Capacitance=1e-6  Setx0=off  InitialVoltage=0  Measurements=None
  L : PMIOPort  Tag=PMCPort  Side=Right
  S : PMIOPort  Port=2  Side=Left
  Isec : Outport
  Vsec : Outport  Port=2
  wires:
  Memory/1 -> Isec/1
  Memory1/1 -> Vsec/1
  N/1 -> "Variable-Ratio Transformer "/1
  " 1"/1 -> Memory/1
  CT/1 -> Display/1, " 1"/1
  PT/1 -> Display1/1, "    "/1
  "    "/1 -> Memory1/1
  connections:
  S/RConn1 -- "Variable-Ratio Transformer "/LConn1
  Ground2/LConn1 -- "Variable-Ratio Transformer "/RConn2
  Ground3/LConn1 -- "Variable-Ratio Transformer "/LConn2
  "Variable-Ratio Transformer "/RConn1 -- rs/LConn1
  CT/RConn1 -- L/RConn1
  PT/LConn1 -- rs/RConn1 -- CT/LConn1
  PT/LConn2 -- Ground1/LConn1

== system IEEE34_PQload/SM_IEEE34/Regulator 1/Single Phase SVR_C/Voltage Regulator Control ==
  note: N= 1/ (1+TapPosition*DeltaU)
  Vm : Inport
  1 : Constant
  Constant : Constant  Value=RegulatorOn
  Constant5 : Constant
  Product : Product  Inputs=/*
  Sum : Sum
  Tap Changer Control : Subsystem  mask(Tap Changer Control){MinMaxTap=TapMinMax, InitialPosition=InitialTap, MecDelay=TapSelectionTime}
      mask prompts: MinMaxTap "Minimum and maximum tap number [ Min  Max ] :"; InitialPosition "Initial tap position"; MecDelay "Mechanical delay time"
      mask init:
      | if MecDelay<=0,
      | 	MecDelay=1/60;
      | end
  Voltage change per tap : Gain  Gain=DeltaU
  Voltage regulator : Subsystem  mask{Vref=RegulatorVref*120, DeadBand=RegulatorDeadBand*120, TimeDelay=RegulatorDelay}
      mask prompts: Vref "Vref (on 120v base)"; DeadBand "Deadband (on 120v base)"; TimeDelay "Time delay (s)"
  N : Outport
  Tap : Outport  Port=2
  wires:
  Vm/1 -> Voltage regulator/1(Vmes (pu))
  Product/1 -> N/1
  Constant/1 -> Voltage regulator/3(RegOn)
  Tap Changer Control/2(Ready) -> Voltage regulator/2(Ready)
  Voltage change per tap/1 -> Sum/2
  Constant5/1 -> Sum/1
  Voltage regulator/1(Up) -> Tap Changer Control/1("Up ")
  Tap Changer Control/1(TapNo) -> Voltage change per tap/1, Tap/1  "Tap"
  1/1 -> Product/2
  Sum/1 -> Product/1
  Voltage regulator/2(Down) -> Tap Changer Control/2("Down ")

== system IEEE34_PQload/SM_IEEE34/Regulator 2/Single Phase SVR_A/Line Drop Compensator ==
  note: Vm=Vsec-Isec(Rc+jXc)
  Isec : Inport
  Vsec : Inport  Port=2
  "        " : spsLinearTransformerLib/Linear Transformer  UNITS=SI  NominalPower=[pNom fNom]  winding1=[vNom/ptRatio 1e-7 1e-8]  winding2=[vNom/ptRatio 1e-7 1e-8]  ThreeWindings=off  winding3=[3.15e+005 0.7938 0.084225]  RmLm=[1e5 1e5]  Measurements=None  DataType=on
  "CTS  " : spsControlledCurrentSourceLib/Controlled Current Source  Initialize=on  Source_Type=AC  Amplitude=0  Phase=0  Frequency=0  Measurements=None
  "PTS  " : spsControlledVoltageSourceLib/Controlled Voltage Source  Initialize=on  Source_Type=AC  Amplitude=0  Phase=0  Frequency=0  Measurements=None
  RMS : spsRMSLib/RMS  TrueRMS=on  Freq=60  RMSInit=120  Ts=0
  Raux : spsSeriesRLCBranchLib/Series RLC Branch  LConnTagsString=__new0  RConnTagsString=__new0  BranchType=R  Resistance=1e2  Inductance=1.6 / (120*pi)  SetiL0=off  InitialCurrent=0  Capacitance=1e-6  Setx0=off  InitialVoltage=0  Measurements=None
  Rc+jXc : spsSeriesRLCBranchLib/Series RLC Branch  LConnTagsString=__new0  RConnTagsString=__new0  BranchType=RL  Resistance=Rc  Inductance=Xc / (2*pi*fNom)  SetiL0=off  InitialCurrent=0  Capacitance=1e-6  Setx0=off  InitialVoltage=0  Measurements=None
  VRelay : spsVoltageMeasurementLib/Voltage Measurement  PhasorSimulation=off  OutputType=Complex  PSBequivalent=0
  Vm : Outport
  wires:
  Vsec/1 -> "PTS  "/1
  Isec/1 -> "CTS  "/1
  VRelay/1 -> RMS/1
  RMS/1 -> Vm/1
  connections:
  VRelay/LConn2 -- "PTS  "/LConn1
  "        "/LConn2 -- "CTS  "/LConn1 -- Raux/RConn1 -- Rc+jXc/RConn1
  "CTS  "/RConn1 -- "        "/LConn1 -- Rc+jXc/LConn1 -- Raux/LConn1
  "        "/RConn2 -- VRelay/LConn1
  "PTS  "/RConn1 -- "        "/RConn1
